simulink model "sg_2d_fir"  (Simulink 7.6)
settings: Solver=ode45  StartTime=0.0  StopTime=1600.0  RelTol=1e-3
undefined symbols (not defined in the file): gcbh, xlBlockLoadCallback, xlGetNormalizedPeriod, xlipgetpartsetting
libraries: xbsIndex_r4 x311, dspsrcs4 x6
(part 2 of 4)

== system sg_2d_fir/sg_2d_fir/5x5_Filters/Green_Filter ==
  Addr : Inport
  Din : Inport  Port=2
  Load : Inport  Port=3
  Coef : Inport  Port=4
  Gain : Inport  Port=5
  5x5_Filter : Subsystem  mask(5x5 Filter){maskNum=Gaussian, coef_n_bits=7, coef_bin_pt=0, gain_n_bits=20, gain_bin_pt=17, smpl_n_bits=8, smpl_bin_pt=0, smpl_period=1, maskCoef=0, maskDiv=0}
      mask prompts: maskNum "5x5 Mask"; coef_n_bits "Coefficient Width"; coef_bin_pt "Coefficient Binary Point"; gain_n_bits "Gain Width"; gain_bin_pt "Gain Binary Point"; smpl_n_bits "Number of Bits per Input Sample"; smpl_bin_pt "Binary Point for Input Samples"; smpl_period "Sample Period"; maskCoef "Mask Value"; maskDiv "Mask Division"
      mask help: The 5x5 Filter block is implemented using 5 n-tap MAC FIR Filters. Nine different 2-D filters have been provided to filter grayscale images.
      mask init: same as sg_2d_fir/sg_2d_fir/5x5_Filters/Blue_Filter/5x5_Filter
      mask StyleString: popup(Identity|Edge|Sobel X|Sobel Y|Sobel X-Y|Blur|Smooth|Sharpen|Gaussian),edit,edit,edit,edit,edit,edit,edit,edit,edit
  Line_Buffer : Subsystem
  Dout : Outport
  wires:
  5x5_Filter/1(Dout) -> Dout/1  "dout"
  Line_Buffer/1(l1) -> 5x5_Filter/1(Line1)  "l1"
  Line_Buffer/2(l2) -> 5x5_Filter/2(Line2)  "l2"
  Line_Buffer/3(l3) -> 5x5_Filter/3(Line3)  "l3"
  Line_Buffer/4(l4) -> 5x5_Filter/4(Line4)  "l4"
  Line_Buffer/5(l5) -> 5x5_Filter/5(Line5)  "l5"
  Din/1 -> Line_Buffer/2(data)  "din"
  Load/1 -> 5x5_Filter/6(load)
  Coef/1 -> 5x5_Filter/7(coef)
  Gain/1 -> 5x5_Filter/8(gain)
  Addr/1 -> Line_Buffer/1(addr)  "addr"

== system sg_2d_fir/sg_2d_fir/5x5_Filters/Red_Filter ==
  Addr : Inport
  Din : Inport  Port=2
  Load : Inport  Port=3
  Coef : Inport  Port=4
  Gain : Inport  Port=5
  5x5_Filter : Subsystem  mask(5x5 Filter){maskNum=Gaussian, coef_n_bits=7, coef_bin_pt=0, gain_n_bits=20, gain_bin_pt=17, smpl_n_bits=8, smpl_bin_pt=0, smpl_period=1, maskCoef=0, maskDiv=0}
      mask prompts: maskNum "5x5 Mask"; coef_n_bits "Coefficient Width"; coef_bin_pt "Coefficient Binary Point"; gain_n_bits "Gain Width"; gain_bin_pt "Gain Binary Point"; smpl_n_bits "Number of Bits per Input Sample"; smpl_bin_pt "Binary Point for Input Samples"; smpl_period "Sample Period"; maskCoef "Mask Value"; maskDiv "Mask Division"
      mask help: The 5x5 Filter block is implemented using 5 n-tap MAC FIR Filters. Nine different 2-D filters have been provided to filter grayscale images.
      mask init: same as sg_2d_fir/sg_2d_fir/5x5_Filters/Blue_Filter/5x5_Filter
      mask StyleString: popup(Identity|Edge|Sobel X|Sobel Y|Sobel X-Y|Blur|Smooth|Sharpen|Gaussian),edit,edit,edit,edit,edit,edit,edit,edit,edit
  Line_Buffer : Subsystem
  Dout : Outport
  wires:
  5x5_Filter/1(Dout) -> Dout/1  "dout"
  Line_Buffer/1(l1) -> 5x5_Filter/1(Line1)  "l1"
  Line_Buffer/2(l2) -> 5x5_Filter/2(Line2)  "l2"
  Line_Buffer/3(l3) -> 5x5_Filter/3(Line3)  "l3"
  Line_Buffer/4(l4) -> 5x5_Filter/4(Line4)  "l4"
  Line_Buffer/5(l5) -> 5x5_Filter/5(Line5)  "l5"
  Din/1 -> Line_Buffer/2(data)  "din"
  Load/1 -> 5x5_Filter/6(load)
  Coef/1 -> 5x5_Filter/7(coef)
  Gain/1 -> 5x5_Filter/8(gain)
  Addr/1 -> Line_Buffer/1(addr)  "addr"

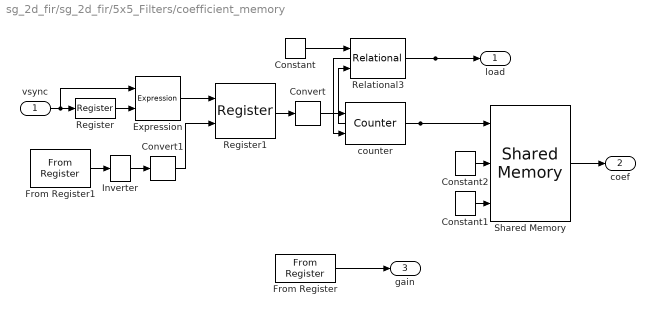
== system sg_2d_fir/sg_2d_fir/5x5_Filters/coefficient_memory ==
  vsync : Inport
  Constant : xbsIndex_r4/Constant  const=25  gui_display_data_type=Fixed-point  arith_type=Unsigned  n_bits=5  bin_pt=0  preci_type=Single  exp_width=8  frac_width=24  explicit_period=on  period=1  equ=P=C  opselect=C  inp2=PCIN>>17  opr=+  inp1=P  carry=CIN  dbl_ovrd=off  block_type=constant
      settings: block_version=10.1.2-Beta
  Constant1 : xbsIndex_r4/Constant  const=0  gui_display_data_type=Fixed-point  arith_type=Boolean  n_bits=width  bin_pt=bin_pt  preci_type=Single  exp_width=8  frac_width=24  explicit_period=off  period=1  equ=P=C  opselect=C  inp2=PCIN>>17  opr=+  inp1=P  carry=CIN  dbl_ovrd=off  block_type=constant
      settings: block_version=VER_STRING_GOES_HERE
  Constant2 : xbsIndex_r4/Constant  const=0  gui_display_data_type=Fixed-point  arith_type=Signed (2's comp)  n_bits=width  bin_pt=bin_pt  preci_type=Single  exp_width=8  frac_width=24  explicit_period=off  period=1  equ=P=C  opselect=C  inp2=PCIN>>17  opr=+  inp1=P  carry=CIN  dbl_ovrd=off  block_type=constant
      settings: block_version=VER_STRING_GOES_HERE
  Convert : xbsIndex_r4/Convert  gui_display_data_type=Fixed-point  arith_type=Boolean  n_bits=1  bin_pt=0  float_type=Single  exp_bits=8  fraction_bits=24  quantization=Truncate  overflow=Wrap  en=off  latency=0  dbl_ovrd=off  pipeline=off  block_type=convert
      settings: block_version=10.1.2-Beta
  Convert1 : xbsIndex_r4/Convert  gui_display_data_type=Fixed-point  arith_type=Boolean  n_bits=1  bin_pt=0  float_type=Single  exp_bits=8  fraction_bits=24  quantization=Truncate  overflow=Wrap  en=off  latency=0  dbl_ovrd=off  pipeline=off  block_type=convert
      settings: block_version=10.1.2-Beta
  Expression : xbsIndex_r4/Expression  expression=~a & b  align_bp=off  en=off  latency=0  precision=Full  arith_type=Unsigned  n_bits=16  bin_pt=0  dbl_ovrd=off  block_type=expr
      settings: block_version=10.1.2-Beta
  From Register : xbsIndex_r4/From Register  shared_memory_name='coef_gain'  init=131072  period=1  ownership=Locally owned and initialized  gui_display_data_type=Fixed-point  arith_type=Unsigned  n_bits=20  bin_pt=17  preci_type=Single  dbl_ovrd=off  block_type=fromreg
      settings: AttributesFormatString=<< %<shared_memory_name> >>  infoedit="Register block that reads data to a shared memory register.  Delay of one sample period."  block_version=10.1
  From Register1 : xbsIndex_r4/From Register  shared_memory_name='coef_update'  init=1  period=1  ownership=Locally owned and initialized  gui_display_data_type=Fixed-point  arith_type=Unsigned  n_bits=1  bin_pt=0  preci_type=Single  dbl_ovrd=off  block_type=fromreg
      settings: AttributesFormatString=<< %<shared_memory_name> >>  infoedit="Register block that reads data to a shared memory register.  Delay of one sample period."  block_version=10.1
  Inverter : xbsIndex_r4/Inverter  en=off  latency=0  dbl_ovrd=off  block_type=inv
      settings: block_version=10.1.2-Beta
  Register : xbsIndex_r4/Register  init=0  rst=off  en=off  dbl_ovrd=off  block_type=register
      settings: block_version=10.1.2-Beta
  Register1 : xbsIndex_r4/Register  init=0  rst=on  en=off  dbl_ovrd=off  block_type=register
      settings: block_version=10.1.2-Beta
  Relational3 : xbsIndex_r4/Relational  mode=a!=b  en=off  latency=0  dbl_ovrd=off  block_type=relational
      settings: block_version=10.1.2-Beta
  Shared Memory : xbsIndex_r4/Shared Memory  shared_memory_name='coef_buffer'  depth=32  ownership=Locally Owned and Initialized  initVector="[0 0 0 0 0  0 0 0 0 0  0 0 1 0 0  0 0 0 0 0  0 0 0 0 0]"  en=off  mutex=Unprotected  mode=Read and Write  write_mode=Read After Write  time_out=0  latency=1  explicit_data_type=on  gui_display_data_type=Fixed-point  arith_type="Signed  (2's comp)"  n_bits=7  bin_pt=0  preci_type=Single  implementation=Block RAM  use_rpm=off  block_type=shmem
      settings: AttributesFormatString=Shared as %<shared_memory_name>  xl_area=[0, 0, 0, 0, 0, 0, 0]  block_version=VER_STRING_GOES_HERE
  counter : xbsIndex_r4/Counter  cnt_type=Count Limited  cnt_to=25  operation=Up  start_count=0  cnt_by_val=1  arith_type=Unsigned  n_bits=5  bin_pt=0  load_pin=off  rst=on  en=on  explicit_period=on  period=period  dbl_ovrd=off  use_behavioral_HDL=off  implementation=Fabric  use_rpm=off  block_type=counter
      settings: infoedit="Configurable up, down and up/down counter.<P><P>Hardware notes: Free running counters are the least expensive in hardware.  A count limited counter is implemented by combining a counter with a comparator."  xl_area=[0, 0, 0, 0, 0, 0, 0]  block_version=VER_STRING_GOES_HERE
  load : Outport
  coef : Outport  Port=2
  gain : Outport  Port=3
  wires:
  Shared Memory/1 -> coef/1
  Constant1/1 -> Shared Memory/3
  counter/1 -> Relational3/2, Shared Memory/1
  Constant2/1 -> Shared Memory/2
  From Register/1 -> gain/1
  Constant/1 -> Relational3/1
  Relational3/1 -> counter/2, load/1
  Convert/1 -> counter/1
  vsync/1 -> Register/1, Expression/1
  Register/1 -> Expression/2
  Register1/1 -> Convert/1
  From Register1/1 -> Inverter/1
  Convert1/1 -> Register1/2
  Expression/1 -> Register1/1
  Inverter/1 -> Convert1/1

== system sg_2d_fir/sg_2d_fir/5x5_Filters/line_ctrs ==
  h : Inport
  rst : Inport  Port=2
  Delay : xbsIndex_r4/Delay  rst=off  infoeditControl=Selection of Reset will increase slice count due to use of real FFs and instead of SRLs  en=off  latency=1  dbl_ovrd=off  reg_retiming=on  block_type=delay
      settings: infoedit="Delay line having  configurable length.<P><P>Hardware notes: A delay line is a chain, each link of which is an SRL16 followed by a flip-flop. If register retiming is enabled, the delay line is a chain of flip-flops."  xl_area=[0, 0, 0, 0, 0, 0, 0]  block_version=VER_STRING_GOES_HERE
  Expression : xbsIndex_r4/Expression  expression=(~d0& d1 ) | rst  align_bp=on  en=off  latency=0  precision=Full  arith_type=Unsigned  n_bits=8  bin_pt=2  dbl_ovrd=off  block_type=expr
      settings: xl_area=[0, 0, 0, 0, 0, 0, 0]  block_version=VER_STRING_GOES_HERE
  Terminator : Terminator
  loop_ctr : Subsystem  mask{nbit=12, init=0, inc=1, limit=4095, stime=1}
      mask prompts: nbit "nbits"; init "initial_value"; inc "increment"; stime "sample time"
      mask help: For ( count=init; count+=inc; count != limit;)
  addr : Outport
  wires:
  Delay/1 -> Expression/2
  loop_ctr/2(tc) -> Terminator/1
  h/1 -> Delay/1, Expression/1
  loop_ctr/1(count) -> addr/1
  rst/1 -> Expression/3
  Expression/1 -> loop_ctr/1(reset)

== system sg_2d_fir/sg_2d_fir/5x5_Filters/Blue_Filter/5x5_Filter ==
  Line1 : Inport
  Line2 : Inport  Port=2
  Line3 : Inport  Port=3
  Line4 : Inport  Port=4
  Line5 : Inport  Port=5
  load : Inport  Port=6
  coef : Inport  Port=7
  gain : Inport  Port=8
  2D_FIR : Subsystem
  load_sequencer : Subsystem  mask{num_coef=length(maskCoef(1,5:-1:1,maskNum))}
      mask prompts: num_coef "Number of Coefficients"
  Dout : Outport
  wires:
  gain/1 -> 2D_FIR/12(gain)
  2D_FIR/1(Dout) -> Dout/1
  load_sequencer/4(load_4) -> 2D_FIR/9(load_4)
  load_sequencer/3(load_3) -> 2D_FIR/8(load_3)
  load_sequencer/2(load_2) -> 2D_FIR/7(load_2)
  load_sequencer/1(load_1) -> 2D_FIR/6(load_1)
  Line3/1 -> 2D_FIR/3(Line3)
  load/1 -> load_sequencer/1(load)
  Line5/1 -> 2D_FIR/5(Line5)
  Line4/1 -> 2D_FIR/4(Line4)
  Line2/1 -> 2D_FIR/2(Line2)
  Line1/1 -> 2D_FIR/1(Line1)
  coef/1 -> 2D_FIR/11(coef)
  load_sequencer/5(load_5) -> 2D_FIR/10(load_5)

== system sg_2d_fir/sg_2d_fir/5x5_Filters/Blue_Filter/Line_Buffer ==
  addr : Inport
  data : Inport  Port=2
  Constant6 : xbsIndex_r4/Constant  const=1  gui_display_data_type=Fixed-point  arith_type=Boolean  n_bits=1  bin_pt=0  preci_type=Single  exp_width=8  frac_width=24  explicit_period=on  period=1  equ=P=C  opselect=C  inp2=PCIN>>17  opr=+  inp1=P  carry=CIN  dbl_ovrd=off  block_type=constant
      settings: block_version=VER_STRING_GOES_HERE
  Delay1 : xbsIndex_r4/Delay  rst=off  infoeditControl=Selection of Reset will increase slice count due to use of real FFs and instead of SRLs  en=off  latency=2  dbl_ovrd=off  reg_retiming=on  block_type=delay
      settings: infoedit="Delay line having  configurable length.<P><P>Hardware notes: A delay line is a chain, each link of which is an SRL16 followed by a flip-flop. If register retiming is enabled, the delay line is a chain of flip-flops."  xl_area=[0, 0, 0, 0, 0, 0, 0]  block_version=VER_STRING_GOES_HERE
  Delay2 : xbsIndex_r4/Delay  rst=off  infoeditControl=Selection of Reset will increase slice count due to use of real FFs and instead of SRLs  en=off  latency=3  dbl_ovrd=off  reg_retiming=on  block_type=delay
      settings: infoedit="Delay line having  configurable length.<P><P>Hardware notes: A delay line is a chain, each link of which is an SRL16 followed by a flip-flop. If register retiming is enabled, the delay line is a chain of flip-flops."  xl_area=[0, 0, 0, 0, 0, 0, 0]  block_version=VER_STRING_GOES_HERE
  Delay7 : xbsIndex_r4/Delay  rst=off  infoeditControl=Selection of Reset will increase slice count due to use of real FFs and instead of SRLs  en=off  latency=4  dbl_ovrd=off  reg_retiming=on  block_type=delay
      settings: infoedit="Delay line having  configurable length.<P><P>Hardware notes: A delay line is a chain, each link of which is an SRL16 followed by a flip-flop. If register retiming is enabled, the delay line is a chain of flip-flops."  xl_area=[0, 0, 0, 0, 0, 0, 0]  block_version=VER_STRING_GOES_HERE
  Delay8 : xbsIndex_r4/Delay  rst=off  infoeditControl=Selection of Reset will increase slice count due to use of real FFs and instead of SRLs  en=off  latency=1  dbl_ovrd=off  reg_retiming=on  block_type=delay
      settings: infoedit="Delay line having  configurable length.<P><P>Hardware notes: A delay line is a chain, each link of which is an SRL16 followed by a flip-flop. If register retiming is enabled, the delay line is a chain of flip-flops."  xl_area=[0, 0, 0, 0, 0, 0, 0]  block_version=VER_STRING_GOES_HERE
  Delay9 : xbsIndex_r4/Delay  rst=off  infoeditControl=Selection of Reset will increase slice count due to use of real FFs and instead of SRLs  en=off  latency=2  dbl_ovrd=off  reg_retiming=on  block_type=delay
      settings: infoedit="Delay line having  configurable length.<P><P>Hardware notes: A delay line is a chain, each link of which is an SRL16 followed by a flip-flop. If register retiming is enabled, the delay line is a chain of flip-flops."  xl_area=[0, 0, 0, 0, 0, 0, 0]  block_version=VER_STRING_GOES_HERE
  Single Port RAM{,1..3} (4 alike) : xbsIndex_r4/Single Port RAM  depth=4096  initVector=0  distributed_mem=Block RAM  write_mode=Read Before Write  rst=off  init_reg=0  en=off  latency=1  dbl_ovrd=off  optimize=Speed  use_rpm=off  block_type=spram
      settings: xl_area=[0, 0, 0, 0, 0, 0, 0]  block_version=8.2
  l1 : Outport
  l2 : Outport  Port=2
  l3 : Outport  Port=3
  l4 : Outport  Port=4
  l5 : Outport  Port=5
  wires:
  Single Port RAM/1 -> Delay8/1, Single Port RAM1/2
  Delay9/1 -> Delay7/1, Single Port RAM3/2
  Single Port RAM1/1 -> l1/1  "l1"
  data/1 -> Delay9/1  "data"
  Delay7/1 -> l5/1  "l5"
  Delay8/1 -> l2/1  "l2"
  Single Port RAM2/1 -> Delay1/1, Single Port RAM/2
  Delay1/1 -> l3/1  "l3"
  Single Port RAM3/1 -> Delay2/1, Single Port RAM2/2
  Delay2/1 -> l4/1  "l4"
  addr/1 -> Single Port RAM3/1, Single Port RAM2/1, Single Port RAM/1, Single Port RAM1/1  "addr"
  Constant6/1 -> Single Port RAM3/3, Single Port RAM2/3, Single Port RAM/3, Single Port RAM1/3

== system sg_2d_fir/sg_2d_fir/5x5_Filters/Ctrl_Delay/Line_Buffer ==
  addr : Inport
  data : Inport  Port=2
  Constant6 : xbsIndex_r4/Constant  const=1  gui_display_data_type=Fixed-point  arith_type=Boolean  n_bits=1  bin_pt=0  preci_type=Single  exp_width=8  frac_width=24  explicit_period=on  period=1  equ=P=C  opselect=C  inp2=PCIN>>17  opr=+  inp1=P  carry=CIN  dbl_ovrd=off  block_type=constant
      settings: block_version=VER_STRING_GOES_HERE
  Delay1 : xbsIndex_r4/Delay  rst=off  infoeditControl=Selection of Reset will increase slice count due to use of real FFs and instead of SRLs  en=off  latency=2  dbl_ovrd=off  reg_retiming=on  block_type=delay
      settings: infoedit="Delay line having  configurable length.<P><P>Hardware notes: A delay line is a chain, each link of which is an SRL16 followed by a flip-flop. If register retiming is enabled, the delay line is a chain of flip-flops."  xl_area=[0, 0, 0, 0, 0, 0, 0]  block_version=VER_STRING_GOES_HERE
  Delay2 : xbsIndex_r4/Delay  rst=off  infoeditControl=Selection of Reset will increase slice count due to use of real FFs and instead of SRLs  en=off  latency=3  dbl_ovrd=off  reg_retiming=on  block_type=delay
      settings: infoedit="Delay line having  configurable length.<P><P>Hardware notes: A delay line is a chain, each link of which is an SRL16 followed by a flip-flop. If register retiming is enabled, the delay line is a chain of flip-flops."  xl_area=[0, 0, 0, 0, 0, 0, 0]  block_version=VER_STRING_GOES_HERE
  Delay7 : xbsIndex_r4/Delay  rst=off  infoeditControl=Selection of Reset will increase slice count due to use of real FFs and instead of SRLs  en=off  latency=4  dbl_ovrd=off  reg_retiming=on  block_type=delay
      settings: infoedit="Delay line having  configurable length.<P><P>Hardware notes: A delay line is a chain, each link of which is an SRL16 followed by a flip-flop. If register retiming is enabled, the delay line is a chain of flip-flops."  xl_area=[0, 0, 0, 0, 0, 0, 0]  block_version=VER_STRING_GOES_HERE
  Delay8 : xbsIndex_r4/Delay  rst=off  infoeditControl=Selection of Reset will increase slice count due to use of real FFs and instead of SRLs  en=off  latency=1  dbl_ovrd=off  reg_retiming=on  block_type=delay
      settings: infoedit="Delay line having  configurable length.<P><P>Hardware notes: A delay line is a chain, each link of which is an SRL16 followed by a flip-flop. If register retiming is enabled, the delay line is a chain of flip-flops."  xl_area=[0, 0, 0, 0, 0, 0, 0]  block_version=VER_STRING_GOES_HERE
  Delay9 : xbsIndex_r4/Delay  rst=off  infoeditControl=Selection of Reset will increase slice count due to use of real FFs and instead of SRLs  en=off  latency=2  dbl_ovrd=off  reg_retiming=on  block_type=delay
      settings: infoedit="Delay line having  configurable length.<P><P>Hardware notes: A delay line is a chain, each link of which is an SRL16 followed by a flip-flop. If register retiming is enabled, the delay line is a chain of flip-flops."  xl_area=[0, 0, 0, 0, 0, 0, 0]  block_version=VER_STRING_GOES_HERE
  Single Port RAM{,1..3} (4 alike) : xbsIndex_r4/Single Port RAM  depth=4096  initVector=0  distributed_mem=Block RAM  write_mode=Read Before Write  rst=off  init_reg=0  en=off  latency=1  dbl_ovrd=off  optimize=Speed  use_rpm=off  block_type=spram
      settings: xl_area=[0, 0, 0, 0, 0, 0, 0]  block_version=8.2
  l1 : Outport
  l2 : Outport  Port=2
  l3 : Outport  Port=3
  l4 : Outport  Port=4
  l5 : Outport  Port=5
  wires:
  Single Port RAM/1 -> Delay8/1, Single Port RAM1/2
  Delay9/1 -> Delay7/1, Single Port RAM3/2
  Single Port RAM1/1 -> l1/1  "l1"
  data/1 -> Delay9/1  "data"
  Delay7/1 -> l5/1  "l5"
  Delay8/1 -> l2/1  "l2"
  Single Port RAM2/1 -> Delay1/1, Single Port RAM/2
  Delay1/1 -> l3/1  "l3"
  Single Port RAM3/1 -> Delay2/1, Single Port RAM2/2
  Delay2/1 -> l4/1  "l4"
  addr/1 -> Single Port RAM3/1, Single Port RAM2/1, Single Port RAM/1, Single Port RAM1/1  "addr"
  Constant6/1 -> Single Port RAM3/3, Single Port RAM2/3, Single Port RAM/3, Single Port RAM1/3

== system sg_2d_fir/sg_2d_fir/5x5_Filters/Green_Filter/5x5_Filter ==
  Line1 : Inport
  Line2 : Inport  Port=2
  Line3 : Inport  Port=3
  Line4 : Inport  Port=4
  Line5 : Inport  Port=5
  load : Inport  Port=6
  coef : Inport  Port=7
  gain : Inport  Port=8
  2D_FIR : Subsystem
  load_sequencer : Subsystem  mask{num_coef=length(maskCoef(1,5:-1:1,maskNum))}
      mask prompts: num_coef "Number of Coefficients"
  Dout : Outport
  wires:
  gain/1 -> 2D_FIR/12(gain)
  2D_FIR/1(Dout) -> Dout/1
  load_sequencer/4(load_4) -> 2D_FIR/9(load_4)
  load_sequencer/3(load_3) -> 2D_FIR/8(load_3)
  load_sequencer/2(load_2) -> 2D_FIR/7(load_2)
  load_sequencer/1(load_1) -> 2D_FIR/6(load_1)
  Line3/1 -> 2D_FIR/3(Line3)
  load/1 -> load_sequencer/1(load)
  Line5/1 -> 2D_FIR/5(Line5)
  Line4/1 -> 2D_FIR/4(Line4)
  Line2/1 -> 2D_FIR/2(Line2)
  Line1/1 -> 2D_FIR/1(Line1)
  coef/1 -> 2D_FIR/11(coef)
  load_sequencer/5(load_5) -> 2D_FIR/10(load_5)

== system sg_2d_fir/sg_2d_fir/5x5_Filters/Green_Filter/Line_Buffer ==
  addr : Inport
  data : Inport  Port=2
  Constant6 : xbsIndex_r4/Constant  const=1  gui_display_data_type=Fixed-point  arith_type=Boolean  n_bits=1  bin_pt=0  preci_type=Single  exp_width=8  frac_width=24  explicit_period=on  period=1  equ=P=C  opselect=C  inp2=PCIN>>17  opr=+  inp1=P  carry=CIN  dbl_ovrd=off  block_type=constant
      settings: block_version=VER_STRING_GOES_HERE
  Delay1 : xbsIndex_r4/Delay  rst=off  infoeditControl=Selection of Reset will increase slice count due to use of real FFs and instead of SRLs  en=off  latency=2  dbl_ovrd=off  reg_retiming=on  block_type=delay
      settings: infoedit="Delay line having  configurable length.<P><P>Hardware notes: A delay line is a chain, each link of which is an SRL16 followed by a flip-flop. If register retiming is enabled, the delay line is a chain of flip-flops."  xl_area=[0, 0, 0, 0, 0, 0, 0]  block_version=VER_STRING_GOES_HERE
  Delay2 : xbsIndex_r4/Delay  rst=off  infoeditControl=Selection of Reset will increase slice count due to use of real FFs and instead of SRLs  en=off  latency=3  dbl_ovrd=off  reg_retiming=on  block_type=delay
      settings: infoedit="Delay line having  configurable length.<P><P>Hardware notes: A delay line is a chain, each link of which is an SRL16 followed by a flip-flop. If register retiming is enabled, the delay line is a chain of flip-flops."  xl_area=[0, 0, 0, 0, 0, 0, 0]  block_version=VER_STRING_GOES_HERE
  Delay7 : xbsIndex_r4/Delay  rst=off  infoeditControl=Selection of Reset will increase slice count due to use of real FFs and instead of SRLs  en=off  latency=4  dbl_ovrd=off  reg_retiming=on  block_type=delay
      settings: infoedit="Delay line having  configurable length.<P><P>Hardware notes: A delay line is a chain, each link of which is an SRL16 followed by a flip-flop. If register retiming is enabled, the delay line is a chain of flip-flops."  xl_area=[0, 0, 0, 0, 0, 0, 0]  block_version=VER_STRING_GOES_HERE
  Delay8 : xbsIndex_r4/Delay  rst=off  infoeditControl=Selection of Reset will increase slice count due to use of real FFs and instead of SRLs  en=off  latency=1  dbl_ovrd=off  reg_retiming=on  block_type=delay
      settings: infoedit="Delay line having  configurable length.<P><P>Hardware notes: A delay line is a chain, each link of which is an SRL16 followed by a flip-flop. If register retiming is enabled, the delay line is a chain of flip-flops."  xl_area=[0, 0, 0, 0, 0, 0, 0]  block_version=VER_STRING_GOES_HERE
  Delay9 : xbsIndex_r4/Delay  rst=off  infoeditControl=Selection of Reset will increase slice count due to use of real FFs and instead of SRLs  en=off  latency=2  dbl_ovrd=off  reg_retiming=on  block_type=delay
      settings: infoedit="Delay line having  configurable length.<P><P>Hardware notes: A delay line is a chain, each link of which is an SRL16 followed by a flip-flop. If register retiming is enabled, the delay line is a chain of flip-flops."  xl_area=[0, 0, 0, 0, 0, 0, 0]  block_version=VER_STRING_GOES_HERE
  Single Port RAM{,1..3} (4 alike) : xbsIndex_r4/Single Port RAM  depth=4096  initVector=0  distributed_mem=Block RAM  write_mode=Read Before Write  rst=off  init_reg=0  en=off  latency=1  dbl_ovrd=off  optimize=Speed  use_rpm=off  block_type=spram
      settings: xl_area=[0, 0, 0, 0, 0, 0, 0]  block_version=8.2
  l1 : Outport
  l2 : Outport  Port=2
  l3 : Outport  Port=3
  l4 : Outport  Port=4
  l5 : Outport  Port=5
  wires:
  Single Port RAM/1 -> Delay8/1, Single Port RAM1/2
  Delay9/1 -> Delay7/1, Single Port RAM3/2
  Single Port RAM1/1 -> l1/1  "l1"
  data/1 -> Delay9/1  "data"
  Delay7/1 -> l5/1  "l5"
  Delay8/1 -> l2/1  "l2"
  Single Port RAM2/1 -> Delay1/1, Single Port RAM/2
  Delay1/1 -> l3/1  "l3"
  Single Port RAM3/1 -> Delay2/1, Single Port RAM2/2
  Delay2/1 -> l4/1  "l4"
  addr/1 -> Single Port RAM3/1, Single Port RAM2/1, Single Port RAM/1, Single Port RAM1/1  "addr"
  Constant6/1 -> Single Port RAM3/3, Single Port RAM2/3, Single Port RAM/3, Single Port RAM1/3

== system sg_2d_fir/sg_2d_fir/5x5_Filters/Red_Filter/5x5_Filter ==
  Line1 : Inport
  Line2 : Inport  Port=2
  Line3 : Inport  Port=3
  Line4 : Inport  Port=4
  Line5 : Inport  Port=5
  load : Inport  Port=6
  coef : Inport  Port=7
  gain : Inport  Port=8
  2D_FIR : Subsystem
  load_sequencer : Subsystem  mask{num_coef=length(maskCoef(1,5:-1:1,maskNum))}
      mask prompts: num_coef "Number of Coefficients"
  Dout : Outport
  wires:
  Line1/1 -> 2D_FIR/1(Line1)
  Line2/1 -> 2D_FIR/2(Line2)
  Line4/1 -> 2D_FIR/4(Line4)
  Line5/1 -> 2D_FIR/5(Line5)
  load/1 -> load_sequencer/1(load)
  Line3/1 -> 2D_FIR/3(Line3)
  load_sequencer/1(load_1) -> 2D_FIR/6(load_1)
  load_sequencer/2(load_2) -> 2D_FIR/7(load_2)
  load_sequencer/3(load_3) -> 2D_FIR/8(load_3)
  load_sequencer/4(load_4) -> 2D_FIR/9(load_4)
  2D_FIR/1(Dout) -> Dout/1
  gain/1 -> 2D_FIR/12(gain)
  coef/1 -> 2D_FIR/11(coef)
  load_sequencer/5(load_5) -> 2D_FIR/10(load_5)

== system sg_2d_fir/sg_2d_fir/5x5_Filters/Red_Filter/Line_Buffer ==
  addr : Inport
  data : Inport  Port=2
  Constant6 : xbsIndex_r4/Constant  const=1  gui_display_data_type=Fixed-point  arith_type=Boolean  n_bits=1  bin_pt=0  preci_type=Single  exp_width=8  frac_width=24  explicit_period=on  period=1  equ=P=C  opselect=C  inp2=PCIN>>17  opr=+  inp1=P  carry=CIN  dbl_ovrd=off  block_type=constant
      settings: block_version=VER_STRING_GOES_HERE
  Delay1 : xbsIndex_r4/Delay  rst=off  infoeditControl=Selection of Reset will increase slice count due to use of real FFs and instead of SRLs  en=off  latency=2  dbl_ovrd=off  reg_retiming=on  block_type=delay
      settings: infoedit="Delay line having  configurable length.<P><P>Hardware notes: A delay line is a chain, each link of which is an SRL16 followed by a flip-flop. If register retiming is enabled, the delay line is a chain of flip-flops."  xl_area=[0, 0, 0, 0, 0, 0, 0]  block_version=VER_STRING_GOES_HERE
  Delay2 : xbsIndex_r4/Delay  rst=off  infoeditControl=Selection of Reset will increase slice count due to use of real FFs and instead of SRLs  en=off  latency=3  dbl_ovrd=off  reg_retiming=on  block_type=delay
      settings: infoedit="Delay line having  configurable length.<P><P>Hardware notes: A delay line is a chain, each link of which is an SRL16 followed by a flip-flop. If register retiming is enabled, the delay line is a chain of flip-flops."  xl_area=[0, 0, 0, 0, 0, 0, 0]  block_version=VER_STRING_GOES_HERE
  Delay7 : xbsIndex_r4/Delay  rst=off  infoeditControl=Selection of Reset will increase slice count due to use of real FFs and instead of SRLs  en=off  latency=4  dbl_ovrd=off  reg_retiming=on  block_type=delay
      settings: infoedit="Delay line having  configurable length.<P><P>Hardware notes: A delay line is a chain, each link of which is an SRL16 followed by a flip-flop. If register retiming is enabled, the delay line is a chain of flip-flops."  xl_area=[0, 0, 0, 0, 0, 0, 0]  block_version=VER_STRING_GOES_HERE
  Delay8 : xbsIndex_r4/Delay  rst=off  infoeditControl=Selection of Reset will increase slice count due to use of real FFs and instead of SRLs  en=off  latency=1  dbl_ovrd=off  reg_retiming=on  block_type=delay
      settings: infoedit="Delay line having  configurable length.<P><P>Hardware notes: A delay line is a chain, each link of which is an SRL16 followed by a flip-flop. If register retiming is enabled, the delay line is a chain of flip-flops."  xl_area=[0, 0, 0, 0, 0, 0, 0]  block_version=VER_STRING_GOES_HERE
  Delay9 : xbsIndex_r4/Delay  rst=off  infoeditControl=Selection of Reset will increase slice count due to use of real FFs and instead of SRLs  en=off  latency=2  dbl_ovrd=off  reg_retiming=on  block_type=delay
      settings: infoedit="Delay line having  configurable length.<P><P>Hardware notes: A delay line is a chain, each link of which is an SRL16 followed by a flip-flop. If register retiming is enabled, the delay line is a chain of flip-flops."  xl_area=[0, 0, 0, 0, 0, 0, 0]  block_version=VER_STRING_GOES_HERE
  Single Port RAM{,1..3} (4 alike) : xbsIndex_r4/Single Port RAM  depth=4096  initVector=0  distributed_mem=Block RAM  write_mode=Read Before Write  rst=off  init_reg=0  en=off  latency=1  dbl_ovrd=off  optimize=Speed  use_rpm=off  block_type=spram
      settings: xl_area=[0, 0, 0, 0, 0, 0, 0]  block_version=8.2
  l1 : Outport
  l2 : Outport  Port=2
  l3 : Outport  Port=3
  l4 : Outport  Port=4
  l5 : Outport  Port=5
  wires:
  Single Port RAM/1 -> Delay8/1, Single Port RAM1/2
  Delay9/1 -> Delay7/1, Single Port RAM3/2
  Single Port RAM1/1 -> l1/1  "l1"
  data/1 -> Delay9/1  "data"
  Delay7/1 -> l5/1  "l5"
  Delay8/1 -> l2/1  "l2"
  Single Port RAM2/1 -> Delay1/1, Single Port RAM/2
  Delay1/1 -> l3/1  "l3"
  Single Port RAM3/1 -> Delay2/1, Single Port RAM2/2
  Delay2/1 -> l4/1  "l4"
  addr/1 -> Single Port RAM3/1, Single Port RAM2/1, Single Port RAM/1, Single Port RAM1/1  "addr"
  Constant6/1 -> Single Port RAM3/3, Single Port RAM2/3, Single Port RAM/3, Single Port RAM1/3

== system sg_2d_fir/sg_2d_fir/5x5_Filters/line_ctrs/loop_ctr ==
  reset : Inport
  AddSub1 : xbsIndex_r4/AddSub  mode=Addition  use_carryin=off  use_carryout=off  en=off  latency=0  precision=User Defined  arith_type=Unsigned  n_bits=nbit  bin_pt=0  quantization=Truncate  overflow=Wrap  dbl_ovrd=off  use_behavioral_HDL=on  hw_selection=Fabric  pipelined=off  use_rpm=off  block_type=addsub
      settings: xl_area=[0, 0, 0, 0, 0, 0, 0]  block_version=VER_STRING_GOES_HERE
  Constant1 : xbsIndex_r4/Constant  const=init-inc  gui_display_data_type=Fixed-point  arith_type=Signed (2's comp)  n_bits=nbit  bin_pt=0  preci_type=Single  exp_width=8  frac_width=24  explicit_period=off  period=1  equ=P=C  opselect=C  inp2=PCIN>>17  opr=+  inp1=P  carry=CIN  dbl_ovrd=off  block_type=constant
      settings: block_version=VER_STRING_GOES_HERE
  Constant6 : xbsIndex_r4/Constant  const=inc  gui_display_data_type=Fixed-point  arith_type=Unsigned  n_bits=nbit  bin_pt=0  preci_type=Single  exp_width=8  frac_width=24  explicit_period=off  period=1  equ=P=C  opselect=C  inp2=PCIN>>17  opr=+  inp1=P  carry=CIN  dbl_ovrd=off  block_type=constant
      settings: block_version=VER_STRING_GOES_HERE
  Constant7 : xbsIndex_r4/Constant  const=floor((limit-init)/inc)*inc-(2*inc)+init  gui_display_data_type=Fixed-point  arith_type=Unsigned  n_bits=nbit  bin_pt=0  preci_type=Single  exp_width=8  frac_width=24  explicit_period=off  period=1  equ=P=C  opselect=C  inp2=PCIN>>17  opr=+  inp1=P  carry=CIN  dbl_ovrd=off  block_type=constant
      settings: block_version=VER_STRING_GOES_HERE
  Expression : xbsIndex_r4/Expression  expression=~(tc | reset)  align_bp=on  en=off  latency=0  precision=Full  arith_type=Unsigned  n_bits=8  bin_pt=2  dbl_ovrd=off  block_type=expr
      settings: xl_area=[0, 0, 0, 0, 0, 0, 0]  block_version=VER_STRING_GOES_HERE
  Mux : xbsIndex_r4/Mux  inputs=2  en=off  latency=0  precision=Full  arith_type="Signed  (2's comp)"  n_bits=8  bin_pt=2  quantization=Truncate  overflow=Wrap  dbl_ovrd=off  block_type=mux
      settings: xl_area=[0, 0, 0, 0, 0, 0, 0]  block_version=VER_STRING_GOES_HERE
  Relational5 : xbsIndex_r4/Relational  mode=a=b  en=off  latency=0  dbl_ovrd=off  block_type=relational
      settings: xl_area=[0, 0, 0, 0, 0, 0, 0]  block_version=VER_STRING_GOES_HERE
  bool : xbsIndex_r4/Convert  gui_display_data_type=Fixed-point  arith_type=Boolean  n_bits=1  bin_pt=0  float_type=Single  exp_bits=8  fraction_bits=24  quantization=Truncate  overflow=Wrap  en=off  latency=0  dbl_ovrd=off  pipeline=off  block_type=convert
      settings: infoedit=The input is presented at the output after quantization and overflow effects.<P><P>Hardware notes: Additional hardware is used when rounding or saturation is selected and output width is less than the input width.  xl_area=[0, 0, 0, 0, 0, 0, 0]  block_version=VER_STRING_GOES_HERE
  bool2 : xbsIndex_r4/Convert  gui_display_data_type=Fixed-point  arith_type="Signed  (2's comp)"  n_bits=nbit+1  bin_pt=0  float_type=Single  exp_bits=8  fraction_bits=24  quantization=Truncate  overflow=Wrap  en=off  latency=0  dbl_ovrd=off  pipeline=off  block_type=convert
      settings: infoedit=The input is presented at the output after quantization and overflow effects.<P><P>Hardware notes: Additional hardware is used when rounding or saturation is selected and output width is less than the input width.  xl_area=[0, 0, 0, 0, 0, 0, 0]  block_version=VER_STRING_GOES_HERE
  rctr : xbsIndex_r4/Register  init=init  rst=off  en=off  dbl_ovrd=off  block_type=register
      settings: xl_area=[0, 0, 0, 0, 0, 0, 0]  block_version=VER_STRING_GOES_HERE
  tcfb1 : xbsIndex_r4/Delay  rst=off  infoeditControl=Selection of Reset will increase slice count due to use of real FFs and instead of SRLs  en=off  latency=1  dbl_ovrd=off  reg_retiming=on  block_type=delay
      settings: infoedit="Delay line having  configurable length.<P><P>Hardware notes: A delay line is a chain, each link of which is an SRL16 followed by a flip-flop. If register retiming is enabled, the delay line is a chain of flip-flops."  xl_area=[0, 0, 0, 0, 0, 0, 0]  block_version=VER_STRING_GOES_HERE
  tcfb2 : xbsIndex_r4/Delay  rst=off  infoeditControl=Selection of Reset will increase slice count due to use of real FFs and instead of SRLs  en=off  latency=1  dbl_ovrd=off  reg_retiming=on  block_type=delay
      settings: infoedit="Delay line having  configurable length.<P><P>Hardware notes: A delay line is a chain, each link of which is an SRL16 followed by a flip-flop. If register retiming is enabled, the delay line is a chain of flip-flops."  xl_area=[0, 0, 0, 0, 0, 0, 0]  block_version=VER_STRING_GOES_HERE
  tco : xbsIndex_r4/Delay  rst=off  infoeditControl=Selection of Reset will increase slice count due to use of real FFs and instead of SRLs  en=off  latency=1  dbl_ovrd=off  reg_retiming=on  block_type=delay
      settings: infoedit="Delay line having  configurable length.<P><P>Hardware notes: A delay line is a chain, each link of which is an SRL16 followed by a flip-flop. If register retiming is enabled, the delay line is a chain of flip-flops."  xl_area=[0, 0, 0, 0, 0, 0, 0]  block_version=VER_STRING_GOES_HERE
  count : Outport
  tc : Outport  Port=2
  wires:
  Constant1/1 -> Mux/2
  AddSub1/1 -> rctr/1
  Constant6/1 -> AddSub1/2
  rctr/1 -> count/1, bool2/1, Relational5/1
  reset/1 -> bool/1
  Expression/1 -> Mux/1
  tco/1 -> tc/1
  Constant7/1 -> Relational5/2
  Relational5/1 -> tcfb1/1
  Mux/1 -> AddSub1/1
  tcfb1/1 -> tco/1, Expression/2
  bool2/1 -> Mux/3
  tcfb2/1 -> Expression/1
  bool/1 -> tcfb2/1

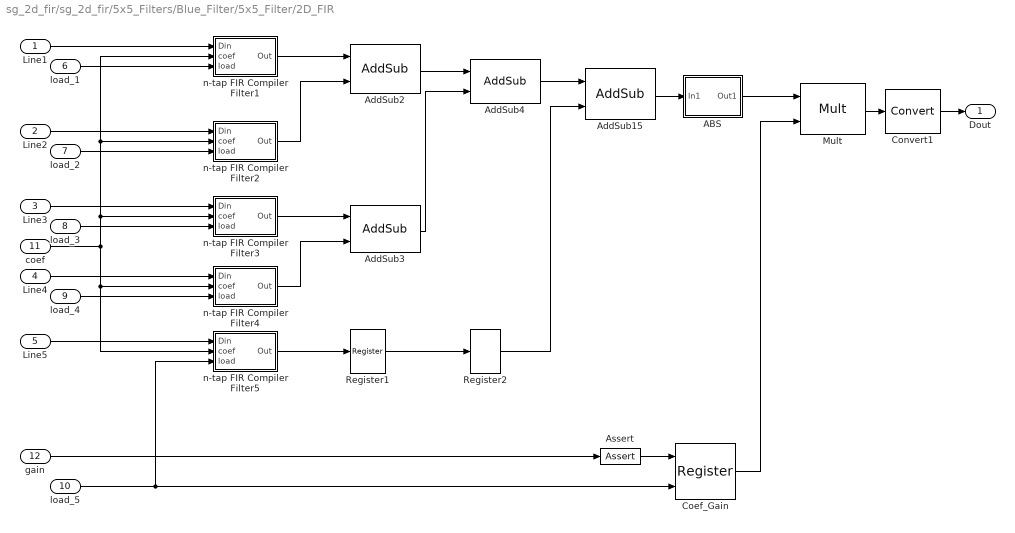
== system sg_2d_fir/sg_2d_fir/5x5_Filters/Blue_Filter/5x5_Filter/2D_FIR ==
  Line1 : Inport
  Line2 : Inport  Port=2
  Line3 : Inport  Port=3
  Line4 : Inport  Port=4
  Line5 : Inport  Port=5
  load_1 : Inport  Port=6
  load_2 : Inport  Port=7
  load_3 : Inport  Port=8
  load_4 : Inport  Port=9
  load_5 : Inport  Port=10
  coef : Inport  Port=11
  gain : Inport  Port=12
  ABS : Subsystem
  AddSub{2..4,15} (4 alike) : xbsIndex_r4/AddSub  mode=Addition  use_carryin=off  use_carryout=off  en=off  latency=1  precision=Full  arith_type=Unsigned  n_bits=8  bin_pt=2  quantization=Truncate  overflow=Wrap  dbl_ovrd=off  use_behavioral_HDL=off  hw_selection=Fabric  pipelined=off  use_rpm=off  block_type=addsub
      settings: xl_area=[0, 0, 0, 0, 0, 0, 0]  block_version=VER_STRING_GOES_HERE
  Assert : xbsIndex_r4/Assert  assert_type=on  type_source=Explicitly  gui_display_data_type=Fixed-point  arith_type=Unsigned  n_bits=gain_n_bits  bin_pt=gain_bin_pt  preci_type=Single  exp_width=8  frac_width=24  assert_rate=off  rate_source=Explicitly  period=1  output_port=on  block_type=assert
      settings: infoedit=Asserts a user-defined sample rate and/or type on a signal.<P><P>Hardware notes: In hardware this block costs nothing.  block_version=9.1.01
  Coef_Gain : xbsIndex_r4/Register  init=0  rst=off  en=on  dbl_ovrd=off  block_type=register
      settings: block_version=9.1.01
  Convert1 : xbsIndex_r4/Convert  gui_display_data_type=Fixed-point  arith_type=Unsigned  n_bits=8  bin_pt=0  float_type=Single  exp_bits=8  fraction_bits=24  quantization=Truncate  overflow=Saturate  en=off  latency=1  dbl_ovrd=off  pipeline=off  block_type=convert
      settings: infoedit=The input is presented at the output after quantization and overflow effects.<P><P>Hardware notes: Additional hardware is used when rounding or saturation is selected and output width is less than the input width.  xl_area=[0, 0, 0, 0, 0, 0, 0]  block_version=VER_STRING_GOES_HERE
  Mult : xbsIndex_r4/Mult  precision=Full  arith_type="Signed  (2's comp)"  n_bits=8  bin_pt=2  quantization=Truncate  overflow=Wrap  en=off  latency=4  dbl_ovrd=off  use_behavioral_HDL=off  opt=Speed  use_embedded=on  optimum_pipeline=off  pipeline=off  use_rpm=off  placement_style=Rectangular shape  block_type=mult
      settings: infoedit=Multiplies two values.<P><P>Hardware notes: To use the internal pipeline stage of the dedicated multiplier you must select 'Pipeline to Greatest Extent Possible'.  xl_area=[0, 0, 0, 0, 0, 0, 0]  block_version=VER_STRING_GOES_HERE
  Register1 : xbsIndex_r4/Register  init=0  rst=off  en=off  dbl_ovrd=off  block_type=register
      settings: xl_area=[0, 0, 0, 0, 0, 0, 0]  block_version=VER_STRING_GOES_HERE
  Register2 : xbsIndex_r4/Register  init=0  rst=off  en=off  dbl_ovrd=off  block_type=register
      settings: xl_area=[0, 0, 0, 0, 0, 0, 0]  block_version=VER_STRING_GOES_HERE
  n-tap FIR Compiler Filter1 : Subsystem  mask{coef=maskCoef(1,5:-1:1,maskNum), coef_n_bits=coef_n_bits, coef_bin_pt=coef_bin_pt}
      mask prompts: coef "Coefficients"; coef_n_bits "Number of Bits per Coefficient"; coef_bin_pt "Binary Point for Coefficients"
      mask help: FIR Compiler based FIR filter with n coefficients
      mask init:
      | dstr = sprintf('%d tap',length(coef));
      | 
      | [bg,fg] = xlcmap('XBlock',0);
      | iPos = get_param(gcb,'Position');
      | iWidth=iPos(3)-iPos(1); iHeight=iPos(4)-iPos(2);
      | iCx=iWidth/2;
      | iCy=iHeight/2;
      | [logoX, logoY] = xlogo(iPos);
      mask Display:
      | patch([0 iWidth iWidth 0],[0 0 iHeight iHeight] , bg);
      | patch(logoX,logoY, fg);
      | text(iCx/1.8,iCy+2,dstr);
      | text(iCx/2.0-4,iCy-10,'FIR Filter');
      | plot([0 0 iWidth iWidth 0], [0 iHeight iHeight 0 0]);
  n-tap FIR Compiler Filter2 : Subsystem  mask{coef=maskCoef(2,5:-1:1,maskNum), coef_n_bits=coef_n_bits, coef_bin_pt=coef_bin_pt}
      mask prompts: coef "Coefficients"; coef_n_bits "Number of Bits per Coefficient"; coef_bin_pt "Binary Point for Coefficients"
      mask help: FIR Compiler based FIR filter with n coefficients
      mask init: same as sg_2d_fir/sg_2d_fir/5x5_Filters/Blue_Filter/5x5_Filter/2D_FIR/n-tap FIR Compiler Filter1
      mask Display:
      | patch([0 iWidth iWidth 0],[0 0 iHeight iHeight] , bg);
      | patch(logoX,logoY, fg);
      | text(iCx/1.8,iCy+2,dstr);
      | text(iCx/2.0-4,iCy-10,'FIR Filter');
      | plot([0 0 iWidth iWidth 0], [0 iHeight iHeight 0 0]);
  n-tap FIR Compiler Filter3 : Subsystem  mask{coef=maskCoef(3,5:-1:1,maskNum), coef_n_bits=coef_n_bits, coef_bin_pt=coef_bin_pt}
      mask prompts: coef "Coefficients"; coef_n_bits "Number of Bits per Coefficient"; coef_bin_pt "Binary Point for Coefficients"
      mask help: FIR Compiler based FIR filter with n coefficients
      mask init: same as sg_2d_fir/sg_2d_fir/5x5_Filters/Blue_Filter/5x5_Filter/2D_FIR/n-tap FIR Compiler Filter1
      mask Display:
      | patch([0 iWidth iWidth 0],[0 0 iHeight iHeight] , bg);
      | patch(logoX,logoY, fg);
      | text(iCx/1.8,iCy+2,dstr);
      | text(iCx/2.0-4,iCy-10,'FIR Filter');
      | plot([0 0 iWidth iWidth 0], [0 iHeight iHeight 0 0]);
  n-tap FIR Compiler Filter4 : Subsystem  mask{coef=maskCoef(4,5:-1:1,maskNum), coef_n_bits=coef_n_bits, coef_bin_pt=coef_bin_pt}
      mask prompts: coef "Coefficients"; coef_n_bits "Number of Bits per Coefficient"; coef_bin_pt "Binary Point for Coefficients"
      mask help: FIR Compiler based FIR filter with n coefficients
      mask init: same as sg_2d_fir/sg_2d_fir/5x5_Filters/Blue_Filter/5x5_Filter/2D_FIR/n-tap FIR Compiler Filter1
      mask Display:
      | patch([0 iWidth iWidth 0],[0 0 iHeight iHeight] , bg);
      | patch(logoX,logoY, fg);
      | text(iCx/1.8,iCy+2,dstr);
      | text(iCx/2.0-4,iCy-10,'FIR Filter');
      | plot([0 0 iWidth iWidth 0], [0 iHeight iHeight 0 0]);
  n-tap FIR Compiler Filter5 : Subsystem  mask{coef=maskCoef(5,5:-1:1,maskNum), coef_n_bits=coef_n_bits, coef_bin_pt=coef_bin_pt}
      mask prompts: coef "Coefficients"; coef_n_bits "Number of Bits per Coefficient"; coef_bin_pt "Binary Point for Coefficients"
      mask help: FIR Compiler based FIR filter with n coefficients
      mask init: same as sg_2d_fir/sg_2d_fir/5x5_Filters/Blue_Filter/5x5_Filter/2D_FIR/n-tap FIR Compiler Filter1
      mask Display:
      | patch([0 iWidth iWidth 0],[0 0 iHeight iHeight] , bg);
      | patch(logoX,logoY, fg);
      | text(iCx/1.8,iCy+2,dstr);
      | text(iCx/2.0-4,iCy-10,'FIR Filter');
      | plot([0 0 iWidth iWidth 0], [0 iHeight iHeight 0 0]);
  Dout : Outport
  wires:
  Assert/1 -> Coef_Gain/1
  coef/1 -> n-tap FIR Compiler Filter5/2(coef), n-tap FIR Compiler Filter4/2(coef), n-tap FIR Compiler Filter3/2(coef), n-tap FIR Compiler Filter2/2(coef), n-tap FIR Compiler Filter1/2(coef)
  load_5/1 -> Coef_Gain/2, n-tap FIR Compiler Filter5/3(load)
  Coef_Gain/1 -> Mult/2
  ABS/1(Out1) -> Mult/1
  Mult/1 -> Convert1/1
  Register2/1 -> AddSub15/2
  AddSub4/1 -> AddSub15/1
  AddSub15/1 -> ABS/1(In1)
  Register1/1 -> Register2/1
  n-tap FIR Compiler Filter5/1(Out) -> Register1/1
  AddSub3/1 -> AddSub4/2
  AddSub2/1 -> AddSub4/1
  n-tap FIR Compiler Filter4/1(Out) -> AddSub3/2
  n-tap FIR Compiler Filter3/1(Out) -> AddSub3/1
  n-tap FIR Compiler Filter2/1(Out) -> AddSub2/2
  n-tap FIR Compiler Filter1/1(Out) -> AddSub2/1
  Line1/1 -> n-tap FIR Compiler Filter1/1(Din)
  load_1/1 -> n-tap FIR Compiler Filter1/3(load)
  Convert1/1 -> Dout/1
  Line2/1 -> n-tap FIR Compiler Filter2/1(Din)
  load_2/1 -> n-tap FIR Compiler Filter2/3(load)
  Line3/1 -> n-tap FIR Compiler Filter3/1(Din)
  load_3/1 -> n-tap FIR Compiler Filter3/3(load)
  Line4/1 -> n-tap FIR Compiler Filter4/1(Din)
  load_4/1 -> n-tap FIR Compiler Filter4/3(load)
  Line5/1 -> n-tap FIR Compiler Filter5/1(Din)
  gain/1 -> Assert/1

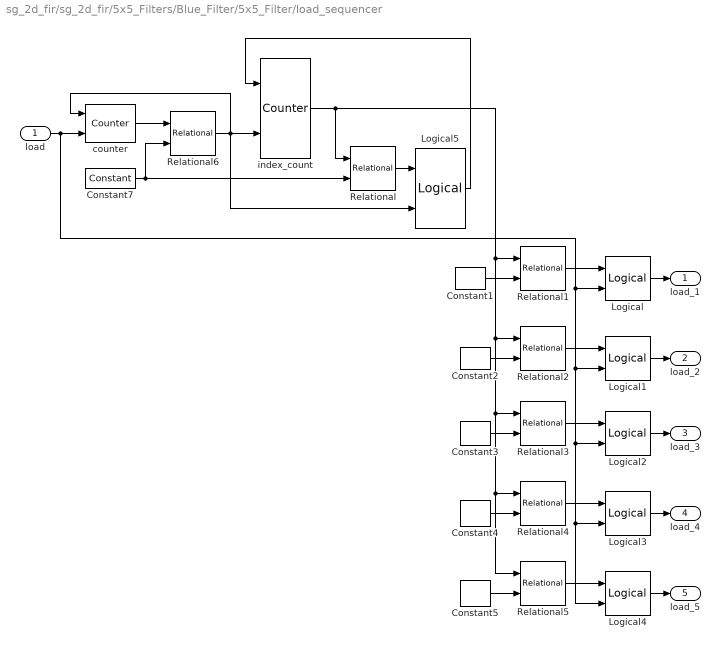
== system sg_2d_fir/sg_2d_fir/5x5_Filters/Blue_Filter/5x5_Filter/load_sequencer ==
  load : Inport
  Constant1 : xbsIndex_r4/Constant  const=0  gui_display_data_type=Fixed-point  arith_type=Unsigned  n_bits=ceil(log2(num_coef))  bin_pt=0  preci_type=Single  exp_width=8  frac_width=24  explicit_period=off  period=1  equ=P=C  opselect=C  inp2=PCIN>>17  opr=+  inp1=P  carry=CIN  dbl_ovrd=off  block_type=constant
      settings: block_version=VER_STRING_GOES_HERE
  Constant2 : xbsIndex_r4/Constant  const=1  gui_display_data_type=Fixed-point  arith_type=Unsigned  n_bits=ceil(log2(num_coef))  bin_pt=0  preci_type=Single  exp_width=8  frac_width=24  explicit_period=off  period=1  equ=P=C  opselect=C  inp2=PCIN>>17  opr=+  inp1=P  carry=CIN  dbl_ovrd=off  block_type=constant
      settings: block_version=VER_STRING_GOES_HERE
  Constant3 : xbsIndex_r4/Constant  const=2  gui_display_data_type=Fixed-point  arith_type=Unsigned  n_bits=ceil(log2(num_coef))  bin_pt=0  preci_type=Single  exp_width=8  frac_width=24  explicit_period=off  period=1  equ=P=C  opselect=C  inp2=PCIN>>17  opr=+  inp1=P  carry=CIN  dbl_ovrd=off  block_type=constant
      settings: block_version=VER_STRING_GOES_HERE
  Constant4 : xbsIndex_r4/Constant  const=3  gui_display_data_type=Fixed-point  arith_type=Unsigned  n_bits=ceil(log2(num_coef))  bin_pt=0  preci_type=Single  exp_width=8  frac_width=24  explicit_period=off  period=1  equ=P=C  opselect=C  inp2=PCIN>>17  opr=+  inp1=P  carry=CIN  dbl_ovrd=off  block_type=constant
      settings: block_version=VER_STRING_GOES_HERE
  Constant5 : xbsIndex_r4/Constant  const=4  gui_display_data_type=Fixed-point  arith_type=Unsigned  n_bits=ceil(log2(num_coef))  bin_pt=0  preci_type=Single  exp_width=8  frac_width=24  explicit_period=off  period=1  equ=P=C  opselect=C  inp2=PCIN>>17  opr=+  inp1=P  carry=CIN  dbl_ovrd=off  block_type=constant
      settings: block_version=VER_STRING_GOES_HERE
  Constant7 : xbsIndex_r4/Constant  const=num_coef-1  gui_display_data_type=Fixed-point  arith_type=Unsigned  n_bits=ceil(log2(num_coef))  bin_pt=0  preci_type=Single  exp_width=8  frac_width=24  explicit_period=off  period=1  equ=P=C  opselect=C  inp2=PCIN>>17  opr=+  inp1=P  carry=CIN  dbl_ovrd=off  block_type=constant
      settings: block_version=VER_STRING_GOES_HERE
  Logical{,1..5} (6 alike) : xbsIndex_r4/Logical  logical_function=AND  inputs=2  en=off  latency=0  precision=Full  arith_type=Unsigned  n_bits=8  bin_pt=2  align_bp=on  dbl_ovrd=off  block_type=logical
      settings: xl_area=[0, 0, 0, 0, 0, 0, 0]  block_version=VER_STRING_GOES_HERE
  Relational{,1..6} (7 alike) : xbsIndex_r4/Relational  mode=a=b  en=off  latency=0  dbl_ovrd=off  block_type=relational
      settings: xl_area=[0, 0, 0, 0, 0, 0, 0]  block_version=VER_STRING_GOES_HERE
  counter : xbsIndex_r4/Counter  cnt_type=Count Limited  cnt_to=num_coef-1  operation=Up  start_count=0  cnt_by_val=1  arith_type=Unsigned  n_bits=ceil(log2(num_coef))  bin_pt=0  load_pin=off  rst=on  en=on  explicit_period=on  period=1  dbl_ovrd=off  use_behavioral_HDL=off  implementation=Fabric  use_rpm=off  block_type=counter
      settings: xl_area=[0, 0, 0, 0, 0, 0, 0]  block_version=VER_STRING_GOES_HERE
  index_count : xbsIndex_r4/Counter  cnt_type=Count Limited  cnt_to=num_coef-1  operation=Up  start_count=0  cnt_by_val=1  arith_type=Unsigned  n_bits=ceil(log2(num_coef))  bin_pt=0  load_pin=off  rst=on  en=on  explicit_period=on  period=1  dbl_ovrd=off  use_behavioral_HDL=off  implementation=Fabric  use_rpm=off  block_type=counter
      settings: infoedit="Configurable up, down and up/down counter.<P><P>Hardware notes: Free running counters are the least expensive in hardware.  A count limited counter is implemented by combining a counter with a comparator."  xl_area=[0, 0, 0, 0, 0, 0, 0]  block_version=VER_STRING_GOES_HERE
  load_1 : Outport
  load_2 : Outport  Port=2
  load_3 : Outport  Port=3
  load_4 : Outport  Port=4
  load_5 : Outport  Port=5
  wires:
  Logical5/1 -> index_count/1
  Relational/1 -> Logical5/1
  index_count/1 -> Relational5/1, Relational4/1, Relational3/1, Relational2/1, Relational1/1, Relational/1
  Relational6/1 -> Logical5/2, counter/1, index_count/2
  Constant7/1 -> Relational/2, Relational6/2
  counter/1 -> Relational6/1
  load/1 -> Logical4/2, Logical3/2, Logical2/2, Logical1/2, Logical/2, counter/2
  Relational5/1 -> Logical4/1
  Logical4/1 -> load_5/1
  Constant5/1 -> Relational5/2
  Relational4/1 -> Logical3/1
  Logical3/1 -> load_4/1
  Constant4/1 -> Relational4/2
  Relational3/1 -> Logical2/1
  Logical2/1 -> load_3/1
  Constant3/1 -> Relational3/2
  Relational2/1 -> Logical1/1
  Logical1/1 -> load_2/1
  Constant2/1 -> Relational2/2
  Logical/1 -> load_1/1
  Relational1/1 -> Logical/1
  Constant1/1 -> Relational1/2
